simulink model "rc1"  (R2018a)
settings: Solver=FixedStepAuto  StartTime=0.0  StopTime=10  FixedStep=1e-5  RelTol=1e-3
settings Model: Creator=user  LastModifiedBy=user

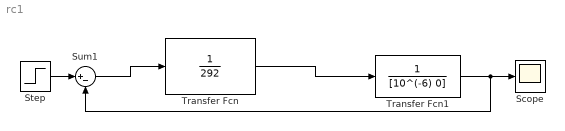
== system rc1 ==
  Scope : Scope
  Step : Step  SampleTime=0
  Sum1 : Sum  Inputs=|+-
  Transfer Fcn : TransferFcn  Denominator=[292]
  Transfer Fcn1 : TransferFcn  Denominator=[10^(-6) 0]
  wires:
  Sum1/1 -> Transfer Fcn/1
  Transfer Fcn/1 -> Transfer Fcn1/1
  Transfer Fcn1/1 -> Scope/1, Sum1/2
  Step/1 -> Sum1/1
